simulink model "PCM"  (R2020b)
settings: Solver=VariableStepAuto  StartTime=0.0  StopTime=10.0  RelTol=1e-3
libraries: commutil2 x1, dspsigops x1, dspquant2 x1
settings Model: Creator=htn  LastModifiedBy=htn

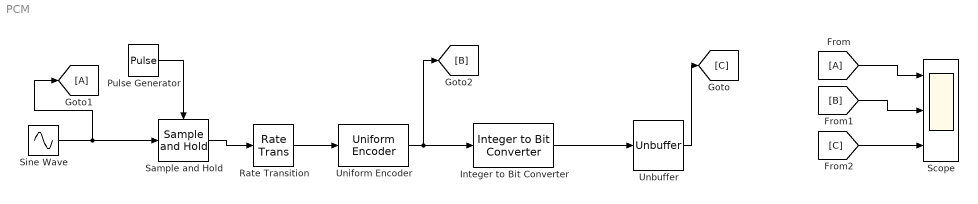
== system PCM ==
  Integer to Bit Converter : commutil2/Integer to Bit Converter  nbits=8  signedInputValues=Unsigned  bitOrder=MSB first  outDtype=Inherit via internal rule
  Pulse Generator : DiscretePulseGenerator  PulseType=Time based  Period=1/8000  PulseWidth=50
  Rate Transition : RateTransition  OutPortSampleTime=1/8000
  Sample and Hold : dspsigops/Sample and Hold  trig=Rising edge  initCond=0  latchinput=off
  Scope : Scope  NumInputPorts=3
  Sine Wave : Sin  Frequency=2*pi*3000  SampleTime=1/64000
  Unbuffer : Unbuffer
  Uniform Encoder : dspquant2/Uniform Encoder  peak=1  bits=8  otype=Unsigned integer
  wires:
  Sine Wave/1 -> [A], Sample and Hold/1
  Unbuffer/1 -> [C]
  Integer to Bit Converter/1 -> Unbuffer/1
  Uniform Encoder/1 -> [B], Integer to Bit Converter/1
  Sample and Hold/1 -> Rate Transition/1
  Rate Transition/1 -> Uniform Encoder/1
  Pulse Generator/1 -> Sample and Hold/Trigger
  [A] -> Scope/1
  [B] -> Scope/2
  [C] -> Scope/3
